simulink model "force_plate_in_VR_v4"  (R2019b)
settings: Solver=ode3  StartTime=0.0  StopTime=inf  FixedStep=0.01  RelTol=1e-3  EnableMultiTasking=on
libraries: mblibv1 x2, xpcrtudplib x1, xpcutilitieslib x1, vrlib x1
settings Model: EnablePacing=on  Creator=kamnikr  LastModifiedBy=student
settings DataIOCC: SaveFormat=Array  SignalLoggingSaveFormat=ModelDataLogs  ReturnWorkspaceOutputs=off
settings OptimizationCC: ExpressionDepthLimit=2147483647  InitFltsAndDblsToZero=on  LifeSpan=inf
settings DebuggingCC: UnderspecifiedInitializationDetection=Classic  MergeDetectMultiDrivingBlocksExec=none  SolverPrmCheckMsg=warning  FcnCallInpInsideContextMsg=warning  StateNameClashWarn=warning  SFUnexpectedBacktrackingDiag=warning  SFNoUnconditionalDefaultTransitionDiag=warning  SFExecutionAtInitializationDiag=none  ArithmeticOperatorsInVariantConditions=warning
settings HardwareCC: ProdBitPerPointer=32  ProdBitPerSizeT=32  ProdBitPerPtrDiffT=32  ProdLargestAtomicFloat=None  ProdIntDivRoundTo=Undefined  ProdEndianess=Unspecified  ProdWordSize=32  ProdHWDeviceType=32-bit Generic
settings ModelReferenceCC: PropagateSignalLabelsOutOfModel=off
settings SFSimCC: SimUseLocalCustomCode=off  CustomCodeUndefinedFunction=UseInterfaceOnly
settings RTWCC: RTWUseLocalCustomCode=off
settings CodeAppCC: StateflowObjectComments=on
settings GRTTargetCC: TargetLangStandard=C89/C90 (ANSI)  GeneratePreprocessorConditionals=Disable all  CombineOutputUpdateFcns=off  GRTInterface=on
settings ConfigComp: CovMetricSettings=dw  CovHtmlReporting=on  CovSaveCumulativeToWorkspaceVar=on  CovSaveSingleToWorkspaceVar=on  CovExternalEMLEnable=off
settings SimscapeCC: SimscapeNormalizeSystem=off

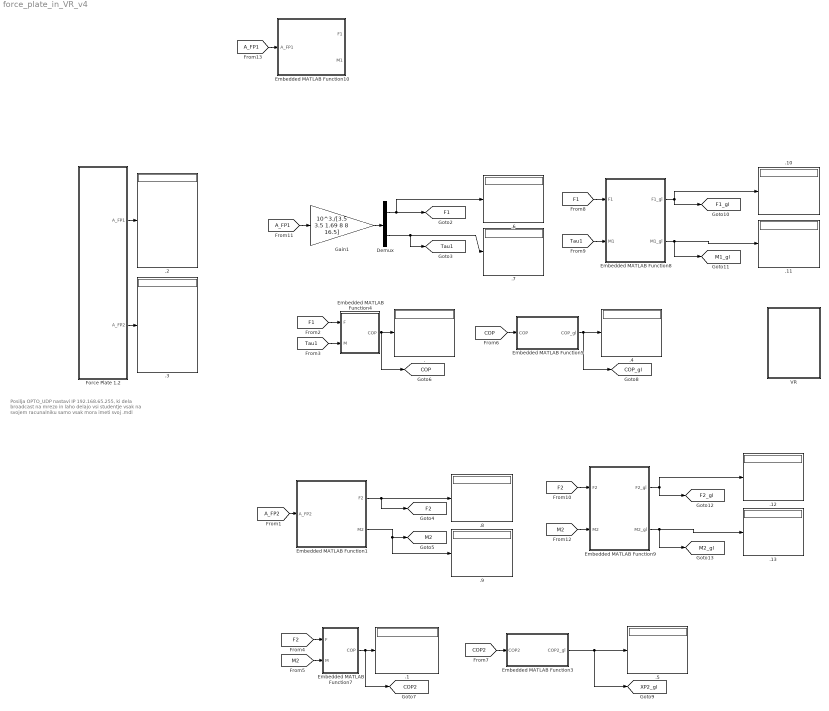
== system force_plate_in_VR_v4 ==
  note: Posilja OPTO_UDP
      | nastavi IP 192.168.65.255, ki dela broadcast na mrezo
      | in laho delajo vsi studentje vsak na svojem racunalniku
      | samo vsak mora imeti svoj .mdl
  .{,1..13} (14 alike) : Display
      settings: Format=bank  Decimation=2
  Demux : Demux  Outputs=[3 3]
  Embedded MATLAB Function1 : MATLAB Function  TreatAsAtomicUnit=on
  Embedded MATLAB Function10 : MATLAB Function  TreatAsAtomicUnit=on
  Embedded MATLAB Function3 : MATLAB Function  TreatAsAtomicUnit=on
  Embedded MATLAB Function4 : MATLAB Function  TreatAsAtomicUnit=on
  Embedded MATLAB Function5 : MATLAB Function  TreatAsAtomicUnit=on
  Embedded MATLAB Function7 : MATLAB Function  TreatAsAtomicUnit=on
  Embedded MATLAB Function8 : MATLAB Function  TreatAsAtomicUnit=on
  Embedded MATLAB Function9 : MATLAB Function  TreatAsAtomicUnit=on
  Force Plate 1,2 : Subsystem
  Gain1 : Gain  Gain=10^3./[3.5 3.5 1.69 8 8 16.5]
  VR : Subsystem
  tag scope: COP2=global, COP=global, COP_gl=global, F1=global, F1_gl=global, F2=global, F2_gl=global, M1_gl=global, M2=global, M2_gl=global, Tau1=global, XP2_gl=global
  wires:
  Force Plate 1,2/1(A_FP1) -> .2/1
  Force Plate 1,2/2(A_FP2) -> .3/1
  [A_FP1] -> Gain1/1
  [A_FP2] -> Embedded MATLAB Function1/1(A_FP2)
  Embedded MATLAB Function4/1(COP) -> ./1, [COP]
  Embedded MATLAB Function7/1(COP) -> .1/1, [COP2]
  [F1] -> Embedded MATLAB Function4/1(F)
  [Tau1] -> Embedded MATLAB Function4/2(M)
  [F2] -> Embedded MATLAB Function7/1(F)
  [M2] -> Embedded MATLAB Function7/2(M)
  [COP] -> Embedded MATLAB Function5/1(COP)
  Embedded MATLAB Function5/1(COP_gl) -> .4/1, [COP_gl]
  [COP2] -> Embedded MATLAB Function3/1(COP2)
  Embedded MATLAB Function3/1(COP2_gl) -> .5/1, [XP2_gl]
  Demux/1 -> .6/1, [F1]
  Demux/2 -> [Tau1], .7/1
  Embedded MATLAB Function1/1(F2) -> .8/1, [F2]
  Embedded MATLAB Function1/2(M2) -> [M2], .9/1
  Embedded MATLAB Function8/1(F1_gl) -> .10/1, [F1_gl]
  Embedded MATLAB Function8/2(M1_gl) -> .11/1, [M1_gl]
  [F1] -> Embedded MATLAB Function8/1(F1)
  [Tau1] -> Embedded MATLAB Function8/2(M1)
  Embedded MATLAB Function9/1(F2_gl) -> .12/1, [F2_gl]
  Embedded MATLAB Function9/2(M2_gl) -> .13/1, [M2_gl]
  [F2] -> Embedded MATLAB Function9/1(F2)
  [M2] -> Embedded MATLAB Function9/2(M2)
  Gain1/1 -> Demux/1
  [A_FP1] -> Embedded MATLAB Function10/1(A_FP1)

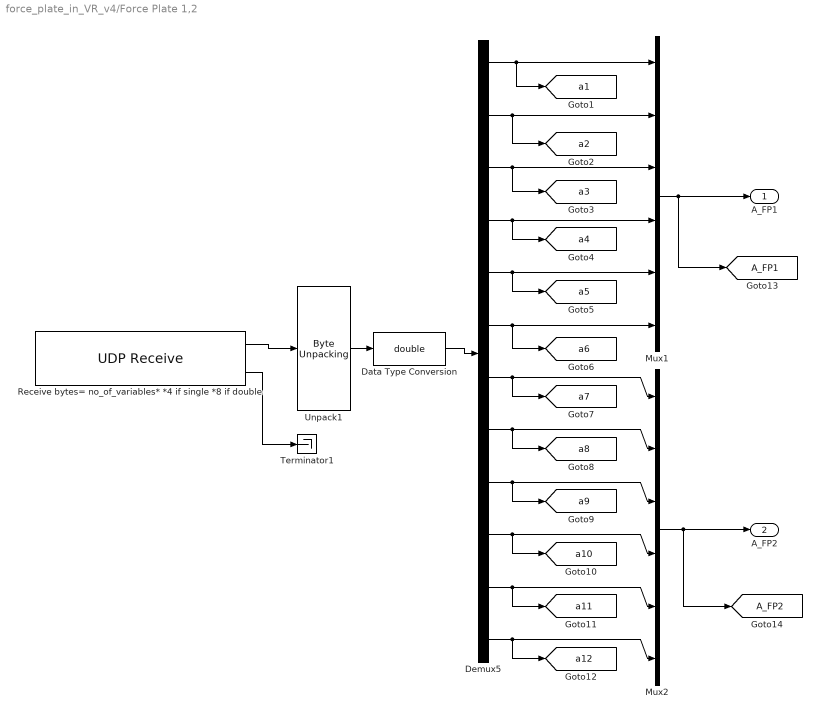
== system force_plate_in_VR_v4/Force Plate 1,2 ==
  Data Type Conversion : DataTypeConversion  OutDataTypeStr=double
  Demux5 : Demux  Outputs=12
  Mux1 : Mux  Inputs=6
  Mux2 : Mux  Inputs=6
  Receive bytes= no_of_variables* *4 if single *8 if double : xpcrtudplib/UDP Receive  ipAddressVal=Use host-target connection  localPort=25001  rcvWidth=(12)*4  rcvFmAny=off  fmAddress=192.168.65.38  rcvMulticast=off  multicastAddress={}  maxUDPQueue=8  sampleTime=0.01
      settings: SourceProductName=Simulink Real-Time
  Terminator1 : Terminator
  Unpack1 : xpcutilitieslib/Byte Unpacking   MaskUnpackedDataTypes={'single'}  MaskUnpackedDataSizes={[1 (12)]}  MaskAlignment=1
      settings: SourceProductName=Simulink Real-Time  SourceProductBaseCode=XP
  A_FP1 : Outport
  A_FP2 : Outport  Port=2
  tag scope: A_FP1=global, A_FP2=global, a10=global, a11=global, a12=global, a1=global, a2=global, a3=global, a4=global, a5=global, a6=global, a7=global, a8=global, a9=global
  wires:
  Receive bytes= no_of_variables* *4 if single *8 if double/1 -> Unpack1/1
  Receive bytes= no_of_variables* *4 if single *8 if double/2 -> Terminator1/1
  Unpack1/1 -> Data Type Conversion/1
  Data Type Conversion/1 -> Demux5/1
  Demux5/1 -> Mux1/1, [a1]
  Demux5/2 -> Mux1/2, [a2]
  Demux5/3 -> Mux1/3, [a3]
  Demux5/4 -> Mux1/4, [a4]
  Demux5/5 -> Mux1/5, [a5]
  Demux5/6 -> Mux1/6, [a6]
  Demux5/7 -> Mux2/1, [a7]
  Demux5/8 -> Mux2/2, [a8]
  Demux5/9 -> Mux2/3, [a9]
  Demux5/10 -> Mux2/4, [a10]
  Demux5/11 -> Mux2/5, [a11]
  Demux5/12 -> Mux2/6, [a12]
  Mux1/1 -> A_FP1/1, [A_FP1]
  Mux2/1 -> A_FP2/1, [A_FP2]

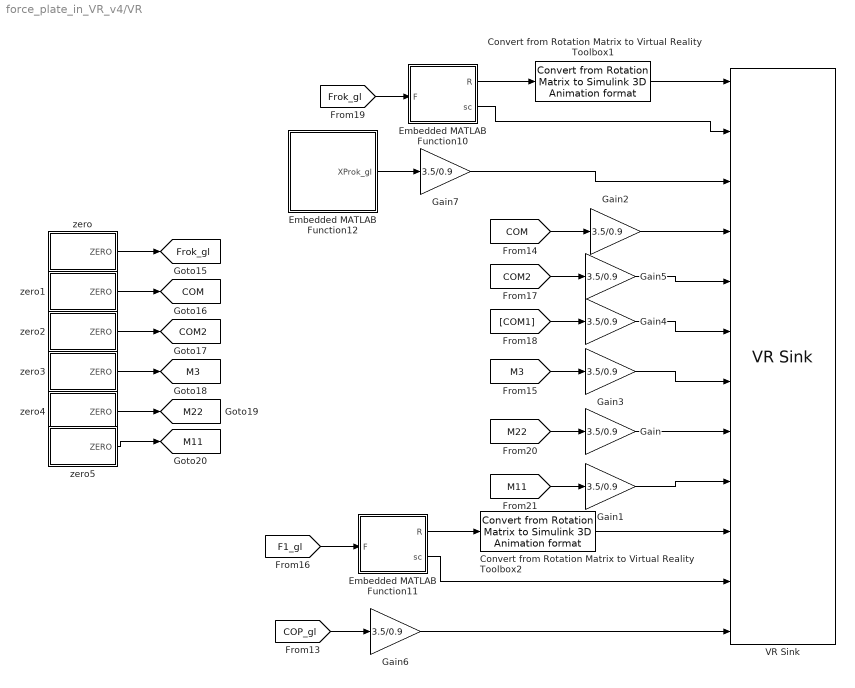
== system force_plate_in_VR_v4/VR ==
  Convert from Rotation Matrix to Virtual Reality Toolbox1 : mblibv1/Utilities/Convert from Rotation Matrix to Simulink 3D Animation format
      settings: SourceProductName=Simscape Multibody  SourceProductBaseCode=MS
  Convert from Rotation Matrix to Virtual Reality Toolbox2 : mblibv1/Utilities/Convert from Rotation Matrix to Simulink 3D Animation format
      settings: SourceProductName=Simscape Multibody  SourceProductBaseCode=MS
  Embedded MATLAB Function10 : MATLAB Function  TreatAsAtomicUnit=on
  Embedded MATLAB Function11 : MATLAB Function  TreatAsAtomicUnit=on
  Embedded MATLAB Function12 : MATLAB Function  TreatAsAtomicUnit=on
  Gain{,1..7} (8 alike) : Gain  Gain=3.5/0.9
  VR Sink : vrlib/VR Sink  InstantiateOnLoad=on  SampleTime=0.01  ViewEnable=on  RemoteChange=off  RemoteView=on  FieldsWritten=Frok_ARROW.rotation.4.1.1.double#Frok_ARROW.scale.3.1.1.double#Frok_ARROW.translation.3.1.1.double#COM.translation.3.1.1.double#COM2.translation.3.1.1.double#COM1.translation.3.1.1.double#M3.translation.3.1.1.double#M2.translation.3.1.1.double#M1.translation.3.1.1.double#F1_ARROW.rotation.4.1.1.double#F1_ARROW.scale.3.1.1.double#F1_ARROW.translation.3.1.1.double  WorldFileName=statika.WRL  WorldDescription=double pendulum  AutoView=off  VideoDimensions=[]  AllowVariableSize=off
      settings: SourceProductName=Simulink
  zero : MATLAB Function  TreatAsAtomicUnit=on
  zero1 : MATLAB Function  TreatAsAtomicUnit=on
  zero2 : MATLAB Function  TreatAsAtomicUnit=on
  zero3 : MATLAB Function  TreatAsAtomicUnit=on
  zero4 : MATLAB Function  TreatAsAtomicUnit=on
  zero5 : MATLAB Function  TreatAsAtomicUnit=on
  tag scope: COM2=global, COM=global, Frok_gl=global, M11=global, M22=global, M3=global
  wires:
  [M22] -> Gain/1
  [M11] -> Gain1/1
  [COM] -> Gain2/1
  [M3] -> Gain3/1
  [COM1] -> Gain4/1
  [COM2] -> Gain5/1
  Embedded MATLAB Function11/1(R) -> Convert from Rotation Matrix to Virtual Reality Toolbox2/1
  [F1_gl] -> Embedded MATLAB Function11/1(F)
  [COP_gl] -> Gain6/1
  Convert from Rotation Matrix to Virtual Reality Toolbox2/1 -> VR Sink/10
  Embedded MATLAB Function11/2(sc) -> VR Sink/11
  Gain6/1 -> VR Sink/12
  Gain1/1 -> VR Sink/9
  Gain/1 -> VR Sink/8
  Gain3/1 -> VR Sink/7
  Gain2/1 -> VR Sink/4
  Gain4/1 -> VR Sink/6
  Gain5/1 -> VR Sink/5
  Embedded MATLAB Function10/1(R) -> Convert from Rotation Matrix to Virtual Reality Toolbox1/1
  [Frok_gl] -> Embedded MATLAB Function10/1(F)
  Embedded MATLAB Function12/1(XProk_gl) -> Gain7/1
  Convert from Rotation Matrix to Virtual Reality Toolbox1/1 -> VR Sink/1
  Embedded MATLAB Function10/2(sc) -> VR Sink/2
  Gain7/1 -> VR Sink/3
  zero/1(ZERO) -> [Frok_gl]
  zero1/1(ZERO) -> [COM]
  zero2/1(ZERO) -> [COM2]
  zero3/1(ZERO) -> [M3]
  zero4/1(ZERO) -> [M22]
  zero5/1(ZERO) -> [M11]

== matlab function force_plate_in_VR_v4/Embedded MATLAB Function1 ==
  data: F2 output; M2 output; A_FP2 input

function [F2,M2] = ReadFP2(A_FP2) 
% This block supports an embeddable subset of the MATLAB language.
% See the help menu for details. 
 

   a7 = A_FP2(1);
   a8 = A_FP2(2);
   a9 = A_FP2(3);
   a10 = A_FP2(4);
   a11 = A_FP2(5);
   a12 = A_FP2(6);




% kalibracija obeh pritiskovnih plosc pretvorba v N in Nm
% load cal.cal
cal =  [2.960, -0.018, -0.009,  0.002, -0.027,  0.041;...
 0.038,  2.997,  0.013, -0.017, -0.008, -0.009;...
 0.052, -0.066, 11.702, -0.115, -0.023,  0.104;...
-0.002,  0.005,  0.002,  1.563, -0.006, -0.010;...
 0.010,  0.000, -0.001,  0.005,  1.556, -0.005;...
-0.014,  0.003,  0.000, -0.003, -0.009,  0.783;...
 2.948,  0.007, -0.001,  0.001, -0.012,  0.001;...
 0.004,  2.989,  0.012,  0.004,  0.004, -0.007;...
-0.148, -0.067, 11.467, -0.006, -0.014, -0.043;...
 0.004, -0.011, -0.001,  1.557,  0.003,  0.005;...
-0.009,  0.001,  0.002, -0.005,  1.542, -0.006;...
 0.001,  0.004, -0.001,  0.006, -0.010,  0.763]; 
 cal=25*cal;

% prva plosca 
% f1=cal(1,1)*a1+cal(1,2)*a2+cal(1,3)*a3+cal(1,4)*a4+cal(1,5)*a5+cal(1,6)*a6;
% f2=cal(2,1)*a1+cal(2,2)*a2+cal(2,3)*a3+cal(2,4)*a4+cal(2,5)*a5+cal(2,6)*a6;
% f3=cal(3,1)*a1+cal(3,2)*a2+cal(3,3)*a3+cal(3,4)*a4+cal(3,5)*a5+cal(3,6)*a6;
% f4=cal(4,1)*a1+cal(4,2)*a2+cal(4,3)*a3+cal(4,4)*a4+cal(4,5)*a5+cal(4,6)*a6;
% f5=cal(5,1)*a1+cal(5,2)*a2+cal(5,3)*a3+cal(5,4)*a4+cal(5,5)*a5+cal(5,6)*a6;
% f6=cal(6,1)*a1+cal(6,2)*a2+cal(6,3)*a3+cal(6,4)*a4+cal(6,5)*a5+cal(6,6)*a6;
% druga plosca
f7=cal(7,1)*a7+cal(7,2)*a8+cal(7,3)*a9+cal(7,4)*a10+cal(7,5)*a11+cal(7,6)*a12;
f8=cal(8,1)*a7+cal(8,2)*a8+cal(8,3)*a9+cal(8,4)*a10+cal(8,5)*a11+cal(8,6)*a12;
f9=cal(9,1)*a7+cal(9,2)*a8+cal(9,3)*a9+cal(9,4)*a10+cal(9,5)*a11+cal(9,6)*a12;
f10=cal(10,1)*a7+cal(10,2)*a8+cal(10,3)*a9+cal(10,4)*a10+cal(10,5)*a11+cal(10,6)*a12;
f11=cal(11,1)*a7+cal(11,2)*a8+cal(11,3)*a9+cal(11,4)*a10+cal(11,5)*a11+cal(11,6)*a12;
f12=cal(12,1)*a7+cal(12,2)*a8+cal(12,3)*a9+cal(12,4)*a10+cal(12,5)*a11+cal(12,6)*a12;
 
  fx2 = f7;
  fy2 = f8;
  fz2 = f9;
  mx2 = f10;
  my2 = f11;
  mz2 = f12;

%butt. filter n=4 za 100Hz s cutoff freq = 10Hz 
%[b,a]=butter(4,10/50);

% fx1=filtfilt(b,a,fx1);
% fy1=filtfilt(b,a,fy1);
% fz1=filtfilt(b,a,fz1);
% mx1=filtfilt(b,a,mx1);
% my1=filtfilt(b,a,my1);
% mz1=filtfilt(b,a,mz1);
%fx2=filtfilt(b,a,fx2);
%fy2=filtfilt(b,a,fy2);
%fz2=filtfilt(b,a,fz2);
%mx2=filtfilt(b,a,mx2);
%my2=filtfilt(b,a,my2);
%mz2=filtfilt(b,a,mz2);  
  
F2 = [fx2 ; fy2; fz2];
M2 = [mx2 ; my2; mz2];
  
  
return;

== matlab function force_plate_in_VR_v4/Embedded MATLAB Function4 ==
  data: COP output; F input; M input
function COP  = COP(F, M)
% This block supports the Embedded MATLAB subset.
% See the help menu for details. 


fx = F(1);
fy = F(2);
fz = F(3);

mx = M(1);
my = M(2);
mz = M(3);


xp = -my/fz;
yp =  mx/fz;
zp = 0;

COP = [xp; yp; zp];

return;

== matlab function force_plate_in_VR_v4/Embedded MATLAB Function7 ==
  data: COP output; F input; M input
function COP  = XP(F, M)
% This block supports the Embedded MATLAB subset.
% See the help menu for details. 


fx = F(1);
fy = F(2);
fz = F(3);

mx = M(1);
my = M(2);
mz = M(3);


xp=(-my/fz);
yp=(mx/fz);
zp=0;

COP = [xp; yp; zp];

return;

== matlab function force_plate_in_VR_v4/Embedded MATLAB Function3 ==
  data: COP2_gl output; COP2 input
function COP2_gl=TransXP(COP2)
% Roman Kamnik


COP2_gl =  rotx(pi/2)*COP2+[0;0;-0.254];  % transformacija za FP2


return;

% %%%%%%%%%%%%%%%%%%%%%%%%%%%%%%%%%%%%%%%%%%%%%%%%%%%%%%%%%%%%%%%%%%%%%%%%%
function c=raz(a,b)

[nr,nc]=size(a);
%if nr==3
   %c=sqrt((a(1,:)-b(1,:)).^2+(a(2,:)-b(2,:)).^2+(a(3,:)-b(3,:)).^2);
   c=sqrt((a(1)-b(1))^2+(a(2)-b(2))^2+(a(3)-b(3))^2);
% elseif nr==2
%      %c=sqrt((a(1,:)-b(1,:)).^2+(a(2,:)-b(2,:)).^2);
%      c=sqrt((a(1)-b(1))^2+(a(2)-b(2))^2);
% end

return; 



%%%%%%%%%%%%%%%%%%%%%%%%%%%%%%%%%%%%%%%%%%%%%%%%%%%%%%%%%%%%%%%%%%%%%%%%

function u = unit(v)
	u = v / norm(v,'fro');
return    


% %%%%%%%%%%%%%%%%%%%%%%%%%%%%%%%%%%%%%%%%%%%%%%%%%%%%%%%%%%%%%%%%%%%%%%%%%
function [e]=envek(v);

[nr,nc]=size(v);

%if nr==3

%e = zeros(1,3);    
%dol=sqrt( v(1,:).^2+v(2,:).^2+v(3,:).^2 );
dol=sqrt( v(1)^2+v(2)^2+v(3)^2);

e(1)=v(1)/dol;
e(2)=v(2)/dol;
e(3)=v(3)/dol;

% elseif nr==2
%    
% dol=sqrt( v(1)^2+v(2)^2 );
% 
% e(1)=v(1)/dol;
% e(2)=v(2)/dol;
% 
% end

return;

% %%%%%%%%%%%%%%%%%%%%%%%%%%%%%%%%%%%%%%%%%%%%%%%%%%%%%%%%%%%%%%%%%%%%%%%%%
function r = rotz(t)
	ct = cos(t);
	st = sin(t);
	r =    [ct	-st	0	
		st	ct	0	
		0	0	1	];
return
% %%%%%%%%%%%%%%%%%%%%%%%%%%%%%%%%%%%%%%%%%%%%%%%%%%%%%%%%%%%%%%%%%%%%%%%%%

function r = rotx(t)
	ct = cos(t);
	st = sin(t);
	r =[1	0	0;...	
		0	ct	-st;...	
		0	st	ct	];
return    
  % %%%%%%%%%%%%%%%%%%%%%%%%%%%%%%%%%%%%%%%%%%%%%%%%%%%%%%%%%%%%%%%%%%%%%%%%%
  
function r = roty(t)
	ct = cos(t);
	st = sin(t);
	r =    [ct	0	st	
            0	1	0	
            -st	0	ct	];
return
% %%%%%%%%%%%%%%%%%%%%%%%%%%%%%%%%%%%%%%%%%%%%%%%%%%%%%%%%%%%%%%%%%%%%%%%%%

== matlab function force_plate_in_VR_v4/Embedded MATLAB Function8 ==
  data: F1 input; M1 input; F1_gl output; M1_gl output
function [F1_gl,M1_gl]= TransFP1(F1, M1) 
% This block supports the Embedded MATLAB subset.
% See the help menu for details. 


% R = [1 0 0 ; 0 1 0 ; 0 0 1 ];

R = rotx(-pi/2)* roty(pi);

F1_gl = R * (-F1);  % transformacija za FP1  

M1_gl = R * (-M1);  % transformacija za FP1 
  
return;


% %%%%%%%%%%%%%%%%%%%%%%%%%%%%%%%%%%%%%%%%%%%%%%%%%%%%%%%%%%%%%%%%%%%%%%%%%
function r = rotz(t)
	ct = cos(t);
	st = sin(t);
	r =    [ct	-st	0	
		st	ct	0	
		0	0	1	];
return
% %%%%%%%%%%%%%%%%%%%%%%%%%%%%%%%%%%%%%%%%%%%%%%%%%%%%%%%%%%%%%%%%%%%%%%%%%

function r = rotx(t)
	ct = cos(t);
	st = sin(t);
	r =[1	0	0;...	
		0	ct	-st;...	
		0	st	ct	];
return    
  % %%%%%%%%%%%%%%%%%%%%%%%%%%%%%%%%%%%%%%%%%%%%%%%%%%%%%%%%%%%%%%%%%%%%%%%%%
  
function r = roty(t)
	ct = cos(t);
	st = sin(t);
	r =    [ct	0	st	
            0	1	0	
            -st	0	ct	];
return
% %%%%%%%%%%%%%%%%%%%%%%%%%%%%%%%%%%%%%%%%%%%%%%%%%%%%%%%%%%%%%%%%%%%%%%%%%

== matlab function force_plate_in_VR_v4/Embedded MATLAB Function9 ==
  data: F2 input; M2 input; F2_gl output; M2_gl output
function [F2_gl,M2_gl]= TransFP1(F2, M2) 
% This block supports the Embedded MATLAB subset.
% See the help menu for details. 


F2_gl = rotx(pi/2)*(-F2);  % transformacija za FP2

M2_gl =  rotx(pi/2)*(-F2);  % transformacija za FP2
  
return;


% %%%%%%%%%%%%%%%%%%%%%%%%%%%%%%%%%%%%%%%%%%%%%%%%%%%%%%%%%%%%%%%%%%%%%%%%%
function r = rotz(t)
	ct = cos(t);
	st = sin(t);
	r =    [ct	-st	0	
		st	ct	0	
		0	0	1	];
return
% %%%%%%%%%%%%%%%%%%%%%%%%%%%%%%%%%%%%%%%%%%%%%%%%%%%%%%%%%%%%%%%%%%%%%%%%%

function r = rotx(t)
	ct = cos(t);
	st = sin(t);
	r =[1	0	0;...	
		0	ct	-st;...	
		0	st	ct	];
return    
  % %%%%%%%%%%%%%%%%%%%%%%%%%%%%%%%%%%%%%%%%%%%%%%%%%%%%%%%%%%%%%%%%%%%%%%%%%
  
function r = roty(t)
	ct = cos(t);
	st = sin(t);
	r =    [ct	0	st	
            0	1	0	
            -st	0	ct	];
return
% %%%%%%%%%%%%%%%%%%%%%%%%%%%%%%%%%%%%%%%%%%%%%%%%%%%%%%%%%%%%%%%%%%%%%%%%%

== matlab function force_plate_in_VR_v4/Embedded MATLAB Function10 ==
  data: F1 output; M1 output; A_FP1 input
function [F1,M1] = ReadFP1(A_FP1) 
% This block supports the Embedded MATLAB subset.
% See the help menu for details. 


   a1 = A_FP1(1);
   a2 = A_FP1(2);
   a3 = A_FP1(3);
   a4 = A_FP1(4);
   a5 = A_FP1(5);
   a6 = A_FP1(6);
   

    FP1offset_0 = 0.0;
    FP1offset_1 = 0.0;
    FP1offset_2 = 0.0;
    FP1offset_3 = 0.0;
    FP1offset_4 = 0.0;
    FP1offset_5 = 0.0;

	v0 =  a1 - FP1offset_0;
	v1 =  a2 - FP1offset_1;
	v2 =  a3 - FP1offset_2;
	v3 =  a4 - FP1offset_3;
	v4 =  a5 - FP1offset_4;
	v5 =  a6 - FP1offset_5;

 CAL0 =2.960  * 25;    CAL1  =-0.018  * 25; CAL2 =-0.009  * 25;  CAL3 =0.002  * 25;   CAL4 =-0.027  * 25;  CAL5 =0.041  * 25;
 CAL6 =0.038  * 25;    CAL7  = 2.997  * 25; CAL8 =0.013  * 25;   CAL9 =-0.017  * 25;  CAL10 =-0.008  * 25; CAL11 =-0.009  * 25;
 CAL12 =0.052  * 25;   CAL13 =-0.066  * 25; CAL14 =11.702  * 25; CAL15 =-0.115  * 25; CAL16 =-0.023  * 25; CAL17 =0.104  * 25;
 CAL18 =-0.002  * 25;  CAL19 =0.005  * 25;  CAL20 =0.002  * 25;  CAL21 =1.563  * 25;  CAL22 =-0.006  * 25; CAL23 =-0.010  * 25;
 CAL24 =0.010  * 25;   CAL25 =0.000  * 25;  CAL26 =-0.001  * 25; CAL27 =0.005  * 25;  CAL28 =1.556  * 25;  CAL29 =-0.005  * 25;
 CAL30 =-0.014  * 25;  CAL31 =0.003  * 25;  CAL32 =0.000  * 25;  CAL33 =-0.003  * 25; CAL34 =-0.009  * 25; CAL35 =0.783  * 25;

 % for (ii = 0; ii <= 35; ii++ 
	% CAL = 25*CAL;

 f1 =CAL0  .*v0 + CAL1  .*v1 + CAL2 .*v2+  CAL3 .*v3 +  CAL4 .*v4  + CAL5 .*v5;
 f2 =CAL6  .*v0 + CAL7  .*v1 + CAL8 .*v2+  CAL9 .*v3 +  CAL10 .*v4 + CAL11 .*v5;
 f3 =CAL12 .*v0 + CAL13 .*v1+ CAL14 .*v2+ CAL15 .*v3 + CAL16 .*v4 + CAL17 .*v5;
 f4 =CAL18 .*v0 + CAL19 .*v1+ CAL20 .*v2+ CAL21 .*v3 + CAL22 .*v4 + CAL23 .*v5;
 f5 =CAL24 .*v0 + CAL25 .*v1+ CAL26 .*v2+ CAL27 .*v3 + CAL28 .*v4 + CAL29 .*v5;
 f6 =CAL30 .*v0 + CAL31 .*v1+ CAL32 .*v2+ CAL33 .*v3 + CAL34 .*v4 + CAL35 .*v5;
 
%   fx1 = -f2;
%   fy1 = -f1;
%   fz1 = -f3;
%   mx1 = -f5;
%   my1 = -f4;
%   mz1 = -f6;
  
  fx1 = f1;
  fy1 = f2;
  fz1 = f3;
  mx1 = f4;
  my1 = f5;
  mz1 = f6;

  F1= [fx1 ; fy1; fz1];
  M1= [mx1 ; my1; mz1];
  
return;

== matlab function force_plate_in_VR_v4/VR/Embedded MATLAB Function10 ==
  data: R output; F input size=[3 1]; sc output
function [R,sc] = fcn1(F)
% This block supports the Embedded MATLAB subset.
% See the help menu for details. 



VERT = [0,1,0]; % vertikala
A = cross(F,VERT);
N = cross(F, A);
O = F;
RR = [unit(N(:)) unit(O(:)) unit(A(:))];  % dolocitev orientacijske R matrike segmenta
%R = [RR(1,1); RR(2,1); RR(3,1); RR(1,2); RR(2,2); RR(3,2); RR(1,3); RR(2,3); RR(3,3)]; % narobe
R = [RR(1,1); RR(1,2); RR(1,3); RR(2,1); RR(2,2); RR(2,3); RR(3,1); RR(3,2); RR(3,3)];



% SKALIRANJE VEKTORJA
%sc = [1;scale;1];

%dolzina vektorja 

d = norm(F);
k = (0.5/800)*(3.5/0.9);  % 0.5 m za 800 N 

sc = [1;d*k;1];



return


function u = unit(v)
	u = v / norm(v,'fro');
return

== matlab function force_plate_in_VR_v4/VR/Embedded MATLAB Function12 ==
  data: XProk_gl output
function XProk_gl  = fcn1
% This block supports the Embedded MATLAB subset.
% See the help menu for details. 

XProk_gl = [0; 0.88; 0]


return;

== matlab function force_plate_in_VR_v4/VR/zero ==
  data: ZERO output
function ZERO  = fcn1
% This block supports the Embedded MATLAB subset.
% See the help menu for details. 

ZERO = [0.0; 0.0; 0];


return;

== matlab function force_plate_in_VR_v4/VR/zero1 ==
  data: ZERO output
function ZERO  = fcn1
% This block supports the Embedded MATLAB subset.
% See the help menu for details. 

ZERO = [0.0; 0.0; 0];


return;

== matlab function force_plate_in_VR_v4/VR/zero2 ==
  data: ZERO output
function ZERO  = fcn1
% This block supports the Embedded MATLAB subset.
% See the help menu for details. 

ZERO = [0.0; 0.0; 0];


return;

== matlab function force_plate_in_VR_v4/Embedded MATLAB Function5 ==
  data: COP_gl output; COP input
function COP_gl=TransCOP(COP)
% Roman Kamnik


% R = [1 0 0 ; 0 1 0 ; 0 0 1 ];
R = rotx(-pi/2)* roty(pi);
COP_gl = R * COP + [0;0;0.254];  % transformacija za FP1


return;

% %%%%%%%%%%%%%%%%%%%%%%%%%%%%%%%%%%%%%%%%%%%%%%%%%%%%%%%%%%%%%%%%%%%%%%%%%
function c=raz(a,b)

[nr,nc]=size(a);
%if nr==3
   %c=sqrt((a(1,:)-b(1,:)).^2+(a(2,:)-b(2,:)).^2+(a(3,:)-b(3,:)).^2);
   c=sqrt((a(1)-b(1))^2+(a(2)-b(2))^2+(a(3)-b(3))^2);
% elseif nr==2
%      %c=sqrt((a(1,:)-b(1,:)).^2+(a(2,:)-b(2,:)).^2);
%      c=sqrt((a(1)-b(1))^2+(a(2)-b(2))^2);
% end

return; 



%%%%%%%%%%%%%%%%%%%%%%%%%%%%%%%%%%%%%%%%%%%%%%%%%%%%%%%%%%%%%%%%%%%%%%%%

function u = unit(v)
	u = v / norm(v,'fro');
return    


% %%%%%%%%%%%%%%%%%%%%%%%%%%%%%%%%%%%%%%%%%%%%%%%%%%%%%%%%%%%%%%%%%%%%%%%%%
function [e]=envek(v);

[nr,nc]=size(v);

%if nr==3

%e = zeros(1,3);    
%dol=sqrt( v(1,:).^2+v(2,:).^2+v(3,:).^2 );
dol=sqrt( v(1)^2+v(2)^2+v(3)^2);

e(1)=v(1)/dol;
e(2)=v(2)/dol;
e(3)=v(3)/dol;

% elseif nr==2
%    
% dol=sqrt( v(1)^2+v(2)^2 );
% 
% e(1)=v(1)/dol;
% e(2)=v(2)/dol;
% 
% end

return;

% %%%%%%%%%%%%%%%%%%%%%%%%%%%%%%%%%%%%%%%%%%%%%%%%%%%%%%%%%%%%%%%%%%%%%%%%%
function r = rotz(t)
	ct = cos(t);
	st = sin(t);
	r =    [ct	-st	0	
		st	ct	0	
		0	0	1	];
return
% %%%%%%%%%%%%%%%%%%%%%%%%%%%%%%%%%%%%%%%%%%%%%%%%%%%%%%%%%%%%%%%%%%%%%%%%%

function r = rotx(t)
	ct = cos(t);
	st = sin(t);
	r =[1	0	0;...	
		0	ct	-st;...	
		0	st	ct	];
return    
  % %%%%%%%%%%%%%%%%%%%%%%%%%%%%%%%%%%%%%%%%%%%%%%%%%%%%%%%%%%%%%%%%%%%%%%%%%
  
function r = roty(t)
	ct = cos(t);
	st = sin(t);
	r =    [ct	0	st	
            0	1	0	
            -st	0	ct	];
return
% %%%%%%%%%%%%%%%%%%%%%%%%%%%%%%%%%%%%%%%%%%%%%%%%%%%%%%%%%%%%%%%%%%%%%%%%%

== matlab function force_plate_in_VR_v4/VR/zero3 ==
  data: ZERO output
function ZERO  = fcn1
% This block supports the Embedded MATLAB subset.
% See the help menu for details. 

ZERO = [0.0; 0.0; 0];


return;

== matlab function force_plate_in_VR_v4/VR/zero4 ==
  data: ZERO output
function ZERO  = fcn1
% This block supports the Embedded MATLAB subset.
% See the help menu for details. 

ZERO = [0.0; 0.0; 0];


return;

== matlab function force_plate_in_VR_v4/VR/zero5 ==
  data: ZERO output
function ZERO  = fcn1
% This block supports the Embedded MATLAB subset.
% See the help menu for details. 

ZERO = [0.0; 0.0; 0];


return;

== matlab function force_plate_in_VR_v4/VR/Embedded MATLAB Function11 ==
  data: R output; F input size=[3 1]; sc output
function [R,sc] = fcn1(F)
% This block supports the Embedded MATLAB subset.
% See the help menu for details. 



VERT = [0,1,0]; % vertikala
A = cross(F,VERT);
N = cross(F, A);
O = F;
RR = [unit(N(:)) unit(O(:)) unit(A(:))];  % dolocitev orientacijske R matrike segmenta
%R = [RR(1,1); RR(2,1); RR(3,1); RR(1,2); RR(2,2); RR(3,2); RR(1,3); RR(2,3); RR(3,3)]; % narobe
R = [RR(1,1); RR(1,2); RR(1,3); RR(2,1); RR(2,2); RR(2,3); RR(3,1); RR(3,2); RR(3,3)];



% SKALIRANJE VEKTORJA
%sc = [1;scale;1];

%dolzina vektorja 

d = norm(F);
k = (0.5/800)*(3.5/0.9);  % 0.5 m za 800 N 

sc = [1;d*k;1];



return


function u = unit(v)
	u = v / norm(v,'fro');
return
